simulink model "PFV_rooftop2Parte2"  (R2017a)
settings: Solver=ode45  StartTime=0.0  StopTime=1  MaxStep=1e-4  RelTol=1e-3
libraries: powerlib x23, simulink x6, re_lib x1, powerlib_meascontrol x1
settings Model: Creator=alfonso  LastModifiedBy=alfonso

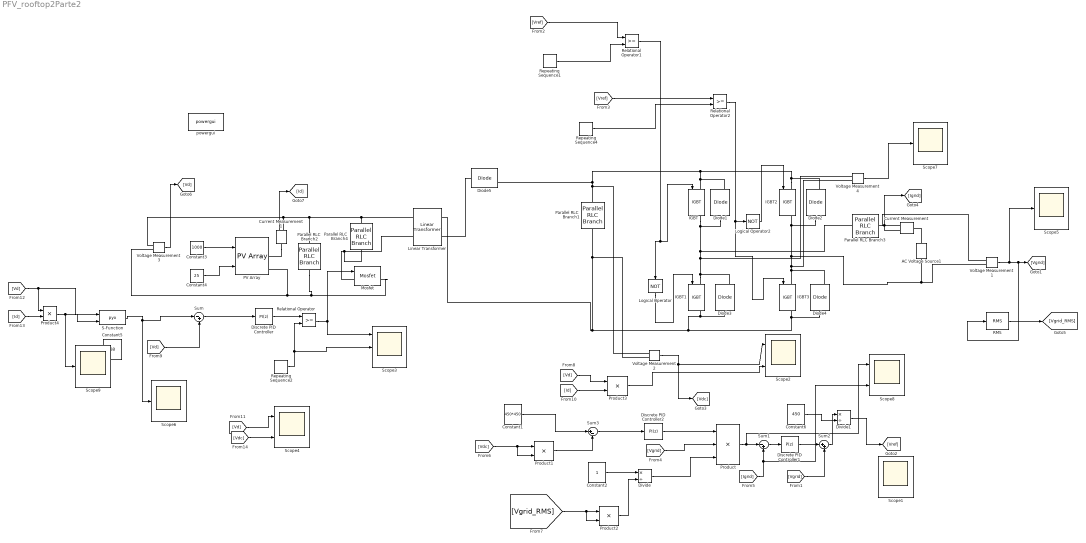
== system PFV_rooftop2Parte2 ==
  AC Voltage Source1 : powerlib/Electrical Sources/AC Voltage Source  Amplitude=230*sqrt(2)  Phase=0  Frequency=50  SampleTime=0  Measurements=None  BusType=swing  Pref=10e3  Qref=0  Qmin=-inf  Qmax=+inf
  Constant1 : Constant  Value=450*450
  Constant2 : Constant
  Constant3 : Constant  Value=1000
  Constant4 : Constant  Value=25
  Constant5 : Constant  Value=68
  Constant6 : Constant  Value=450
  Current Measurement : powerlib/Measurements/Current Measurement  PhasorSimulation=off  OutputType=Complex  PSBequivalent=0
  Current Measurement1 : powerlib/Measurements/Current Measurement  PhasorSimulation=off  OutputType=Complex  PSBequivalent=0
  Diode{1..5} (5 alike) : powerlib/Power Electronics/Diode  Ron=0.001  Lon=0  Vf=0.8  IC=0  UseSnubber=0  Rs=500  Cs=250e-9  Measurements=on
  Discrete PID Controller : simulink/Continuous/PID Controller  Controller=PI  TimeDomain=Discrete-time  SampleTime=1e-4  IntegratorMethod=Forward Euler  FilterMethod=Forward Euler  Form=Parallel  UseFilter=on  ControllerParametersSource=internal  P=2e-3  I=2  D=0  N=100  InitialConditionSource=internal  InitialConditionForIntegrator=0  InitialConditionForFilter=0  ExternalReset=none  LimitOutput=off  UpperSaturationLimit=inf  LowerSaturationLimit=-inf  LinearizeAsGain=off  AntiWindupMode=none  Kb=1  TrackingMode=off  Kt=1  PParamMin=[]  PParamMax=[]  IParamMin=[]  IParamMax=[]  DParamMin=[]  DParamMax=[]  NParamMin=[]  NParamMax=[]  KbParamMin=[]  KbParamMax=[]  KtParamMin=[]  KtParamMax=[]  POutMin=[]  POutMax=[]  IOutMin=[]  IOutMax=[]  DOutMin=[]  DOutMax=[]  NOutMin=[]  NOutMax=[]  KbOutMin=[]  KbOutMax=[]  KtOutMin=[]  KtOutMax=[]  IntegratorOutMin=[]  IntegratorOutMax=[]  FilterOutMin=[]  FilterOutMax=[]  SumOutMin=[]  SumOutMax=[]  SumI1OutMin=[]  SumI1OutMax=[]  SumI2OutMin=[]  SumI2OutMax=[]  SumI3OutMin=[]  SumI3OutMax=[]  SumDOutMin=[]  SumDOutMax=[]  SaturationOutMin=[]  SaturationOutMax=[]  IntegratorContinuousStateAttributes=''  IntegratorStateMustResolveToSignalObject=off  IntegratorRTWStateStorageClass=Auto  FilterContinuousStateAttributes=''  FilterStateMustResolveToSignalObject=off  FilterRTWStateStorageClass=Auto  DifferentiatorICPrevScaledInput=0  DifferentiatorOutMin=[]  DifferentiatorOutMax=[]  InitialConditionSetting=State (most efficient)
  Discrete PID Controller1 : simulink/Continuous/PID Controller  Controller=P  TimeDomain=Discrete-time  SampleTime=1e-4  IntegratorMethod=Forward Euler  FilterMethod=Forward Euler  Form=Parallel  UseFilter=on  ControllerParametersSource=internal  P=1e3  I=10  D=0  N=100  InitialConditionSource=internal  InitialConditionForIntegrator=0  InitialConditionForFilter=0  ExternalReset=none  LimitOutput=off  UpperSaturationLimit=inf  LowerSaturationLimit=-inf  LinearizeAsGain=off  AntiWindupMode=none  Kb=1  TrackingMode=off  Kt=1  PParamMin=[]  PParamMax=[]  IParamMin=[]  IParamMax=[]  DParamMin=[]  DParamMax=[]  NParamMin=[]  NParamMax=[]  KbParamMin=[]  KbParamMax=[]  KtParamMin=[]  KtParamMax=[]  POutMin=[]  POutMax=[]  IOutMin=[]  IOutMax=[]  DOutMin=[]  DOutMax=[]  NOutMin=[]  NOutMax=[]  KbOutMin=[]  KbOutMax=[]  KtOutMin=[]  KtOutMax=[]  IntegratorOutMin=[]  IntegratorOutMax=[]  FilterOutMin=[]  FilterOutMax=[]  SumOutMin=[]  SumOutMax=[]  SumI1OutMin=[]  SumI1OutMax=[]  SumI2OutMin=[]  SumI2OutMax=[]  SumI3OutMin=[]  SumI3OutMax=[]  SumDOutMin=[]  SumDOutMax=[]  SaturationOutMin=[]  SaturationOutMax=[]  IntegratorContinuousStateAttributes=''  IntegratorStateMustResolveToSignalObject=off  IntegratorRTWStateStorageClass=Auto  FilterContinuousStateAttributes=''  FilterStateMustResolveToSignalObject=off  FilterRTWStateStorageClass=Auto  DifferentiatorICPrevScaledInput=0  DifferentiatorOutMin=[]  DifferentiatorOutMax=[]  InitialConditionSetting=State (most efficient)
  Discrete PID Controller2 : simulink/Continuous/PID Controller  Controller=PI  TimeDomain=Discrete-time  SampleTime=1e-4  IntegratorMethod=Forward Euler  FilterMethod=Forward Euler  Form=Parallel  UseFilter=on  ControllerParametersSource=internal  P=5e-3  I=5e-2  D=0  N=100  InitialConditionSource=internal  InitialConditionForIntegrator=0  InitialConditionForFilter=0  ExternalReset=none  LimitOutput=off  UpperSaturationLimit=inf  LowerSaturationLimit=-inf  LinearizeAsGain=off  AntiWindupMode=none  Kb=1  TrackingMode=off  Kt=1  PParamMin=[]  PParamMax=[]  IParamMin=[]  IParamMax=[]  DParamMin=[]  DParamMax=[]  NParamMin=[]  NParamMax=[]  KbParamMin=[]  KbParamMax=[]  KtParamMin=[]  KtParamMax=[]  POutMin=[]  POutMax=[]  IOutMin=[]  IOutMax=[]  DOutMin=[]  DOutMax=[]  NOutMin=[]  NOutMax=[]  KbOutMin=[]  KbOutMax=[]  KtOutMin=[]  KtOutMax=[]  IntegratorOutMin=[]  IntegratorOutMax=[]  FilterOutMin=[]  FilterOutMax=[]  SumOutMin=[]  SumOutMax=[]  SumI1OutMin=[]  SumI1OutMax=[]  SumI2OutMin=[]  SumI2OutMax=[]  SumI3OutMin=[]  SumI3OutMax=[]  SumDOutMin=[]  SumDOutMax=[]  SaturationOutMin=[]  SaturationOutMax=[]  IntegratorContinuousStateAttributes=''  IntegratorStateMustResolveToSignalObject=off  IntegratorRTWStateStorageClass=Auto  FilterContinuousStateAttributes=''  FilterStateMustResolveToSignalObject=off  FilterRTWStateStorageClass=Auto  DifferentiatorICPrevScaledInput=0  DifferentiatorOutMin=[]  DifferentiatorOutMax=[]  InitialConditionSetting=State (most efficient)
  Divide : Product  Inputs=*/
  Divide1 : Product  Inputs=*/
  IGBT{,1..3} (4 alike) : powerlib/Power Electronics/IGBT  Ron=0.001  Lon=0  Vf=1  Tf=1e-6  Tt=2e-6  IC=0  Rs=1e5  Cs=inf  Measurements=on
  Linear Transformer : powerlib/Elements/Linear Transformer  UNITS=SI  NominalPower=[ 500 50 ]  winding1=[60 0 0]  winding2=[450 0 0]  ThreeWindings=off  winding3=[3.15e+05 315.06 0.12769]  RmLm=[2.3346e+09 0]  Measurements=Winding currents  DataType=on
  Logical Operator : Logic  Operator=NOT  AllPortsSameDT=off  OutDataTypeStr=boolean
  Logical Operator2 : Logic  Operator=NOT  AllPortsSameDT=off  OutDataTypeStr=boolean
  Mosfet : powerlib/Power Electronics/Mosfet  Ron=0.1  Lon=0  Rd=0.01  Vfd=0  IC=0  Rs=1e5  Cs=inf  Measurements=on
  PV Array : re_lib/Solar/PV Array  Npar=1  Nser=2  PlotType=array @ 1000 W/m2 & specified temperatures  S_vec="[ 1000  500  100 ]"  Temp_C_vec="[ 45 25  ]"  ModuleName=1Soltech 1STH-215-P  PlotWhenSelected=off  Pm=213.15  Ncell=60  Voc=36.3  Isc=7.84  Vm=29  Im=7.35  beta_Voc_pc=-0.36099  alpha_Isc_pc=0.102  beta_Voc=-0.13104  alpha_Isc=0.007997  IL=7.8649  I0=2.9259e-10  nI=0.98117  Rsh=313.3991  Rs=0.39383  BAL=off  Tc=1e-6  Tfilter=5e-5
  Parallel RLC Branch1 : powerlib/Elements/Parallel RLC Branch  LConnTagsString=a  RConnTagsString=__new0  BranchType=C  Resistance=1  Inductance=5e-2  SetiL0=off  InitialCurrent=0  Capacitance=1e-3  Setx0=off  InitialVoltage=0  Measurements=None
  Parallel RLC Branch2 : powerlib/Elements/Parallel RLC Branch  LConnTagsString=a  RConnTagsString=__new0  BranchType=C  Resistance=1  Inductance=5e-3  SetiL0=off  InitialCurrent=0  Capacitance=5e-3  Setx0=off  InitialVoltage=0  Measurements=None
  Parallel RLC Branch3 : powerlib/Elements/Parallel RLC Branch  LConnTagsString=a  RConnTagsString=__new0  BranchType=L  Resistance=1  Inductance=5e-3  SetiL0=off  InitialCurrent=0  Capacitance=1.5e-2  Setx0=off  InitialVoltage=0  Measurements=None
  Parallel RLC Branch4 : powerlib/Elements/Parallel RLC Branch  LConnTagsString=a  RConnTagsString=__new0  BranchType=L  Resistance=1  Inductance=5e-3  SetiL0=off  InitialCurrent=0  Capacitance=1.5e-2  Setx0=off  InitialVoltage=0  Measurements=None
  Product : Product  Inputs=3
  Product{1..4} (4 alike) : Product
  RMS : powerlib_meascontrol/Measurements/RMS  TrueRMS=on  Freq=60  RMSInit=120  Ts=0
  Relational Operator : RelationalOperator  OutDataTypeStr=boolean  RndMeth=Simplest
  Relational Operator1 : RelationalOperator  OutDataTypeStr=boolean  RndMeth=Simplest
  Relational Operator2 : RelationalOperator  OutDataTypeStr=boolean  RndMeth=Simplest
  Repeating Sequence1 : simulink/Sources/Repeating Sequence  rep_seq_t=[0 50e-06 100e-06]  rep_seq_y=[-1 1 -1]
  Repeating Sequence2 : simulink/Sources/Repeating Sequence  rep_seq_t=[0 1/10000]  rep_seq_y=[0 1]
  Repeating Sequence4 : simulink/Sources/Repeating Sequence  rep_seq_t=[0 50e-06 100e-06]  rep_seq_y=[1 -1 1]
  S-Function : S-Function  FunctionName=pyo  SFunctionDeploymentMode=off  EnableBusSupport=off
  Scope{1,5..7,9} (5 alike) : Scope
  Scope2 : Scope  NumInputPorts=2
  Scope3 : Scope  NumInputPorts=3
  Scope4 : Scope  NumInputPorts=2
  Scope8 : Scope  NumInputPorts=2
  Sum : Sum  Inputs=|-+
  Sum1 : Sum  Inputs=|-+
  Sum2 : Sum  Inputs=|++
  Sum3 : Sum  Inputs=|+-
  Voltage Measurement{1..4} (4 alike) : powerlib/Measurements/Voltage Measurement  PhasorSimulation=off  OutputType=Complex  PSBequivalent=0
  powergui : powerlib/powergui  Priority=1  SimulationMode=Discrete  SampleTime=1e-6  frequency=60  Iterations=50  frequencyindice=0  Pbase=100e6  ErrMax=1e-4  UnitsV=kV  UnitsW=MW  buscounter=0  FunctionMessages=off  echomessages=off  EnableUseOfTLC=off  CurrentSourceSwitches=off  DisableSnubberDevices=off  DisableRonSwitches=off  DisableVfSwitches=off  DisplayEquations=off  SolverType=Tustin/Backward Euler (TBE)  Interpol=off  ExternalGateDelay=off  methode=off  Ts=100  x0status=blocks  SPID=on  SwTol=0  HookPort=off  RestoreLinks=warning  ResistiveCurrentMeasurement=off  Frange=[0:2:500]  Ylog=off  Xlog=on  ShowGrid=off  save=off  variable=ZData  structure=0  ZoomFFT=off  StartTime=0.0  cycles=1  DisplayStyle=1  fundamental=60  FreqAxis=off  MaxFrequency=1000  frequencyindicesteady=1  RmsSteady=1  display=off
  wires:
  [Vref] -> Relational Operator2/1
  Sum1/1 -> Discrete PID Controller1/1
  [Igrid] -> Scope8/2, Sum1/2
  Divide/1 -> Product/3
  Discrete PID Controller2/1 -> Product/1
  Relational Operator2/1 -> IGBT3/1, Logical Operator2/1
  Repeating Sequence4/1 -> Relational Operator2/2
  [Vref] -> Relational Operator1/1
  Repeating Sequence1/1 -> Relational Operator1/2
  [Vgrid] -> Product/2
  Voltage Measurement1/1 -> Scope5/1, RMS/1, [Vgrid]
  Product/1 -> Scope8/1, Sum1/1
  Relational Operator1/1 -> Logical Operator/1, IGBT/1
  Current Measurement/1 -> [Igrid]
  Logical Operator/1 -> IGBT1/1
  Logical Operator2/1 -> IGBT2/1
  Discrete PID Controller1/1 -> Sum2/1
  [Vgrid] -> Sum2/2
  Voltage Measurement2/1 -> [Vdc], Scope2/1
  Sum3/1 -> Discrete PID Controller2/1
  [Vdc] -> Product1/2, Product1/1
  Product1/1 -> Sum3/2
  RMS/1 -> [Vgrid_RMS]
  [Vgrid_RMS] -> Product2/2, Product2/1
  Product2/1 -> Divide/2
  Constant2/1 -> Divide/1
  Constant1/1 -> Sum3/1
  Constant3/1 -> PV Array/1
  Relational Operator/1 -> Scope3/1, Mosfet/1
  Repeating Sequence2/1 -> Scope3/2, Relational Operator/2
  Current Measurement1/1 -> [Id]
  Constant4/1 -> PV Array/2
  Voltage Measurement3/1 -> [Vd]
  [Vd] -> Sum/2
  Discrete PID Controller/1 -> Relational Operator/1
  [Vd] -> Product3/1
  [Id] -> Product3/2
  Product3/1 -> Scope2/2
  [Vd] -> Scope4/1
  [Id] -> Product4/2
  Product4/1 -> Scope9/1, S-Function/2
  [Vd] -> Product4/1, S-Function/1
  S-Function/1 -> Sum/1, Scope6/1
  Voltage Measurement4/1 -> Scope7/1
  Sum/1 -> Discrete PID Controller/1
  [Vdc] -> Scope4/2
  Constant6/1 -> Divide1/2
  Sum2/1 -> Divide1/1
  Divide1/1 -> [Vref]
  connections:
  IGBT3/RConn1 -- Diode4/LConn1 -- Linear Transformer/RConn1 -- Voltage Measurement2/LConn2 -- Parallel RLC Branch1/RConn1 -- Diode3/LConn1 -- IGBT1/RConn1
  IGBT1/LConn1 -- Voltage Measurement4/LConn1 -- Diode1/LConn1 -- IGBT/RConn1 -- Parallel RLC Branch3/LConn1 -- Diode3/RConn1
  Voltage Measurement1/LConn2 -- AC Voltage Source1/LConn1 -- Diode2/LConn1 -- IGBT2/RConn1 -- Voltage Measurement4/LConn2 -- Diode4/RConn1 -- IGBT3/LConn1
  Parallel RLC Branch3/RConn1 -- Voltage Measurement1/LConn1 -- Current Measurement/RConn1
  IGBT2/LConn1 -- Diode2/RConn1 -- Diode5/RConn1 -- Voltage Measurement2/LConn1 -- Parallel RLC Branch1/LConn1 -- Diode1/RConn1 -- IGBT/LConn1
  AC Voltage Source1/RConn1 -- Current Measurement/LConn1
  Current Measurement1/RConn1 -- Voltage Measurement3/LConn1 -- Parallel RLC Branch2/LConn1 -- Linear Transformer/LConn1 -- Parallel RLC Branch4/RConn1
  Mosfet/RConn1 -- Parallel RLC Branch2/RConn1 -- PV Array/RConn2 -- Voltage Measurement3/LConn2
  Parallel RLC Branch4/LConn1 -- Linear Transformer/LConn2 -- Mosfet/LConn1
  Current Measurement1/LConn1 -- PV Array/RConn1
  Linear Transformer/RConn2 -- Diode5/LConn1
